simulink model "stm32f4_data_logger_ascii_demo"  (Simulink 7.3)
settings: Solver=FixedStepDiscrete  SolverMode=SingleTasking  StartTime=0.0  StopTime=10.0  RelTol=1e-3
PreLoadFcn:
  | waijung.modelPreload; % Required for working with Waijung Blockset. Do not remove.
undefined symbols (not defined in the file): HSEOSC, Link, LQFP176, ST, STM32F417IG
libraries: simulink x3, stm32f4_sdio_lib x1, stm32f4_io_lib x1, stm32f4_adc_lib x1, stm32f4_device_config_lib x1
CloseFcn:
  | waijung.modelClose; % Required for working with Waijung Blockset. Do not remove.
settings Model: Creator=Krisada  LastModifiedBy=Krisada
settings OptimizationCC: OptimizeModelRefInitCode=on  LifeSpan=1
settings HardwareCC: ProdEndianess=LittleEndian  ProdHWDeviceType=ARM Compatible->Cortex - M4  TargetEndianess=LittleEndian  TargetHWDeviceType=ARM Compatible->Cortex - M4
settings RTWCC: SystemTargetFile=stm32f4.tlc  GenerateMakefile=off  TemplateMakefile=ert_default_tmf  Description=STM32F4 Target  ProcessScript=stm32f4_make_rtw_hook
settings CodeAppCC: IgnoreCustomStorageClasses=off
settings STFCustomTargetCC: ModelReferenceCompliant=off  CombineOutputUpdateFcns=on  ERTCustomFileBanners=on  SupportContinuousTime=off  SupportNonInlinedSFcns=off  SystemTargetFile=stm32f4.tlc
settings ERTTargetCC: MultiwordLength=2048  ModelReferenceCompliant=off  ParMdlRefBuildCompliant=off  CompOptLevelCompliant=off  ERTFirstTimeCompliant=off  ModelStepFunctionPrototypeControlCompliant=off  CPPClassGenCompliant=off  ExtModeMexFile=noextcomm  InlinedParameterPlacement=NonHierarchical  ERTSrcFileBannerTemplate=stm32f4_code_template.cgt  ERTHdrFileBannerTemplate=stm32f4_code_template.cgt  ERTDataSrcFileTemplate=stm32f4_code_template.cgt  ERTDataHdrFileTemplate=stm32f4_code_template.cgt  ERTCustomFileTemplate=stm32f4_file_process.tlc

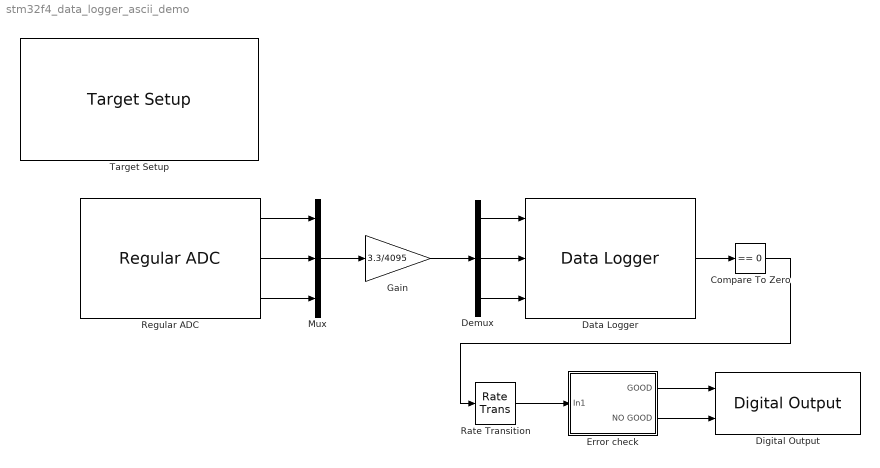
== system stm32f4_data_logger_ascii_demo ==
  Compare To Zero : simulink/Logic and Bit Operations/Compare To Zero  SystemSampleTime=-1  relop===  LogicOutDataTypeMode=uint8  ZeroCross=off
  Data Logger : stm32f4_sdio_lib/Data Logger  variablefilename=off  filename='data.csv'  conf=DataLogger  transfer=Blocking  packet=Ascii  header='data1,data2,data3\r\n'  asciiformat='%f,%f,%f,\r\n'  porttype_double=2  porttype_single=0  porttype_int8=0  porttype_uint8=1  porttype_int16=0  porttype_uint16=0  porttype_int32=0  porttype_uint32=0  advance=off  buffersize=1024  safeprintf=off  createfileoptions=Rename  synctimer=1  enablestatus=on  portpinstr=0  sampletime=-1  blockid=DataLogger  inputporttype=[-1,-1,-1]  inputportwidth=[1,1,1]  inputportlabel={'D0 (single)','D1 (single)','D2 (single)'}  outputporttype=[3]  outputportwidth=[1]  outputportlabel={'Status'}  compat=0  optionstring="[\"on\",\"off\",\"data.csv\",\"Ascii\",\"1024\",\"?\",\"?\",\"off\",\"1000000\",\"Rename\",\"-\",\"-\",\"-\",\"-\",\"-\",\"float\",\"float\",\"float\"]"
  Demux : Demux  Outputs=3
  Digital Output : stm32f4_io_lib/Digital Output  use_bitband=on  port=D  speed=100  porttype=Push Pull  porttypestr=PP  use_pin0=off  use_pin1=off  use_pin2=off  use_pin3=off  use_pin4=off  use_pin5=off  use_pin6=off  use_pin7=off  use_pin8=off  use_pin9=off  use_pin10=off  use_pin11=off  use_pin12=on  use_pin13=on  use_pin14=off  use_pin15=off  pinstr=GPIO_Pin_12 | GPIO_Pin_13  usedpinarray="[0  0  0  0  0  0  0  0  0  0  0  0  1  1  0  0]"  bitbandingstr=|  sampletime=-1  sampletimestr=0.1  blockid=DigitalOutput  enablecustomportlabel=off  globalinit=off  cinputportlabel=In1, In2  coutputportlabel=0
      | #define DigitalOutput_D12 Peripheral_BB(GPIOD->ODR, 12)  /* Output pin */
      | #define DigitalOutput_D13 Peripheral_BB(GPIOD->ODR, 13)  /* Output pin */
  Error check : Subsystem
  Gain : Gain  Gain=3.3/4095  ParameterDataType=fixdt(1, 16)  ParameterScaling=2^0  OutDataType=fixdt(1, 16)  OutScaling=2^0  OutDataTypeStr=Inherit: Same as input  ParamDataTypeStr=Inherit: Same as input
  Mux : Mux  Inputs=3
  Rate Transition : RateTransition  OutPortSampleTime=0.1
  Regular ADC : stm32f4_adc_lib/Regular ADC  adcmodule=1  outputdatatype=Single  prescaler=2  prescalerstr=ADC_Prescaler_Div2  chsamplingtime=Auto  chsamplingtimestr=ADC_SampleTime_480Cycles  read_an0=off  read_an1=off  read_an2=off  read_an3=off  read_an4=off  read_an5=on  read_an6=on  read_an7=on  read_an8=off  read_an9=off  read_an10=off  read_an11=off  read_an12=off  read_an13=off  read_an14=off  read_an15=off  read_an16=off  read_an17=off  read_an18=off  pinstr=GPIO_Pin_5 | GPIO_Pin_6 | GPIO_Pin_7  usedpinarray="[0  0  0  0  0  1  1  1  0  0  0  0  0  0  0  0  0  0  0]"  usedportidarray="[0  0  0]"  usedpinidarray="[5  6  7]"  usedpinidcount=3  sampletime=0.5  blockid=RegularADC  enablecustomportlabel=off  cinputportlabel=0  coutputportlabel=Out1, Out2
  Target Setup : stm32f4_device_config_lib/Target Setup  Priority=100  compiler=GNU ARM  previous_compiler=GNU ARM  mcu=STM32F417IG (LQFP176)  mcustr=STM32F417IG  clockconfig=HSEOSC-8MHz  system_stm32f4xx_c_path=F:\trunk\targets\stm32f4_target\stm32f4\utils\system_stm32f4xx_default\STM32F40_41xxx\hseosc8mhz  showmemoryconfiguration=off  stacksize=0x2000  heapsize=0x2000  enableautocompiledownload=on  fullchiperase=off  programmerinterface=ST-Link  editctrlstr=on  compilercontrolstr=$(patsubst %, -I%, .) -mcpu=cortex-m4 -mthumb -mthumb-interwork -mfloat-abi=hard -mfpu=fpv4-sp-d16 -ffast-math -Wall -Wextra -Ofast  assemblercontrolstr=$(patsubst %, -I%, .) -mcpu=cortex-m4 -mthumb -mthumb-interwork -mfloat-abi=hard -mfpu=fpv4-sp-d16 -ffast-math -Wall -Wextra -Ofast -Wa,-amhls=$(<:.s=.lst) -D__STACK_SIZE=$(STACK_SIZE) -D__HEAP_SIZE=$(HEAP_SIZE)  linkercontrolstr=-T$(LD_SCRIPT) -g -Wl,-Map=$(MAP),--cref,--no-warn-mismatch -mcpu=cortex-m4 -mthumb -mthumb-interwork -mfloat-abi=hard -mfpu=fpv4-sp-d16 -specs=nosys.specs  runafterdownload=on  execprofile=None  profileruart=3  profilerbaud=500000  profilertxpin=D8  profilerinitstr=0.01,168000000,1680000,500000,0  manualsetsampletime=off  sampletime=0.01  blockid=TargetSetup  systickreloadvalue=1680000  hseval=8000000  lastprofileruart=3  hclk=168000000  flashorigin=0x8000000  flashlength=1024k  ramorigin=0x20000000  ramlength=128k  useextram=off
  wires:
  Data Logger/1 -> Compare To Zero/1
  Compare To Zero/1 -> Rate Transition/1
  Error check/1(GOOD) -> Digital Output/1
  Error check/2(NO GOOD) -> Digital Output/2
  Rate Transition/1 -> Error check/1(In1)
  Gain/1 -> Demux/1
  Demux/2 -> Data Logger/2
  Demux/3 -> Data Logger/3
  Demux/1 -> Data Logger/1
  Mux/1 -> Gain/1
  Regular ADC/2 -> Mux/2
  Regular ADC/1 -> Mux/1
  Regular ADC/3 -> Mux/3

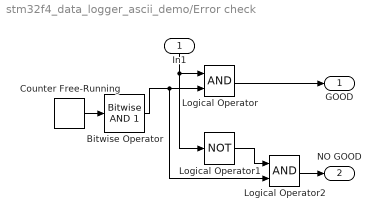
== system stm32f4_data_logger_ascii_demo/Error check ==
  In1 : Inport
  Bitwise Operator : simulink/Logic and Bit Operations/Bitwise Operator  logicop=AND  UseBitMask=on  BitMask=1  BitMaskRealWorld=Stored Integer
  Counter Free-Running : simulink/Sources/Counter Free-Running  SystemSampleTime=-1  NumBits=16  tsamp=-1
  Logical Operator : Logic  AllPortsSameDT=off  OutDataTypeMode=boolean  LogicDataType=fixdt(0, 8)  OutDataTypeStr=boolean
  Logical Operator1 : Logic  Operator=NOT  AllPortsSameDT=off  OutDataTypeMode=boolean  LogicDataType=fixdt(0, 8)  OutDataTypeStr=boolean
  Logical Operator2 : Logic  AllPortsSameDT=off  OutDataTypeMode=boolean  LogicDataType=fixdt(0, 8)  OutDataTypeStr=boolean
  GOOD : Outport
  NO GOOD : Outport  Port=2
  wires:
  In1/1 -> Logical Operator1/1, Logical Operator/1
  Bitwise Operator/1 -> Logical Operator/2, Logical Operator2/2
  Logical Operator1/1 -> Logical Operator2/1
  Counter Free-Running/1 -> Bitwise Operator/1
  Logical Operator/1 -> GOOD/1
  Logical Operator2/1 -> NO GOOD/1
